simulink model "Z_N1"  (R2021b)
settings: Solver=VariableStepAuto  StartTime=0.0  StopTime=100  RelTol=1e-3
settings Model: Creator=Duván Ramírez Lotta  LastModifiedBy=Duván Ramírez Lotta

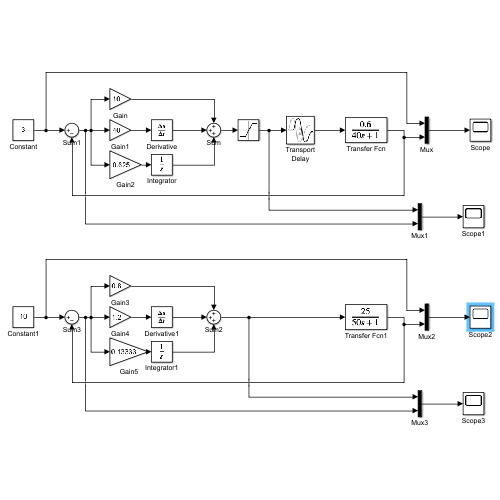
[thumbnail: Simulink's stored preview of the top-level diagram]
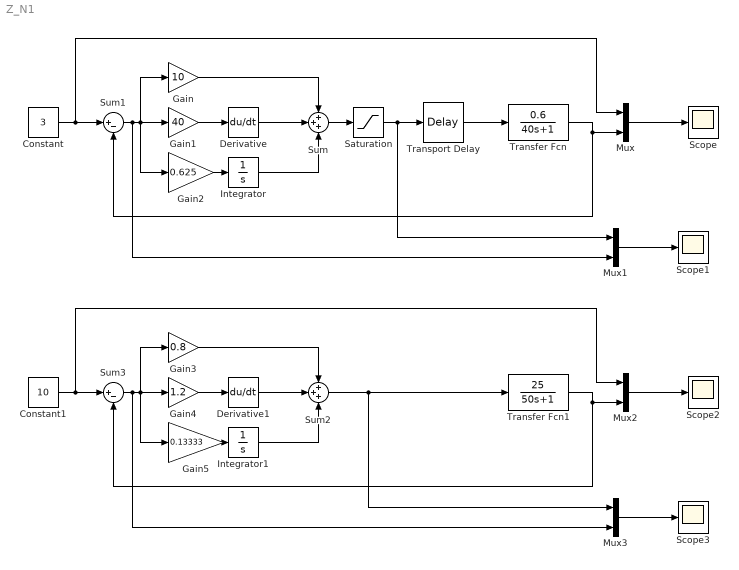
== system Z_N1 ==
  Constant : Constant  Value=3
  Constant1 : Constant  Value=10
  Derivative : Derivative
  Derivative1 : Derivative
  Gain : Gain  Gain=10
  Gain1 : Gain  Gain=40
  Gain2 : Gain  Gain=0.625
  Gain3 : Gain  Gain=0.8
  Gain4 : Gain  Gain=1.2
  Gain5 : Gain  Gain=0.13333
  Integrator : Integrator
  Integrator1 : Integrator
  Mux{,1..3} (4 alike) : Mux  Inputs=2
  Saturation : Saturate  UpperLimit=5  LowerLimit=0
  Scope{,1..3} (4 alike) : Scope
  Sum : Sum  Inputs=+++
  Sum1 : Sum  Inputs=|+-
  Sum2 : Sum  Inputs=+++
  Sum3 : Sum  Inputs=|+-
  Transfer Fcn : TransferFcn  Numerator=0.6  Denominator=[40 1]
  Transfer Fcn1 : TransferFcn  Numerator=25  Denominator=[50 1]
  Transport Delay : TransportDelay  DelayTime=8
  wires:
  Gain1/1 -> Derivative/1
  Gain2/1 -> Integrator/1
  Sum1/1 -> Mux1/2, Gain2/1, Gain/1, Gain1/1
  Derivative/1 -> Sum/2
  Gain/1 -> Sum/1
  Integrator/1 -> Sum/3
  Constant/1 -> Mux/1, Sum1/1
  Transfer Fcn/1 -> Mux/2, Sum1/2
  Transport Delay/1 -> Transfer Fcn/1
  Sum/1 -> Saturation/1
  Mux/1 -> Scope/1
  Mux1/1 -> Scope1/1
  Saturation/1 -> Mux1/1, Transport Delay/1
  Integrator1/1 -> Sum2/3
  Constant1/1 -> Mux2/1, Sum3/1
  Derivative1/1 -> Sum2/2
  Sum3/1 -> Mux3/2, Gain5/1, Gain3/1, Gain4/1
  Mux3/1 -> Scope3/1
  Gain4/1 -> Derivative1/1
  Gain3/1 -> Sum2/1
  Gain5/1 -> Integrator1/1
  Mux2/1 -> Scope2/1
  Transfer Fcn1/1 -> Mux2/2, Sum3/2
  Sum2/1 -> Mux3/1, Transfer Fcn1/1
